simulink library "HORTISIM"  (R2021a)
settings: Solver=VariableStepAuto  StartTime=0.0  StopTime=10.0  RelTol=1e-3
undefined symbols (not defined in the file or in its folder): crop_params, heat_ic, heat_p, p_climate, params_fruit, scr_p, substrate_params, tp_tilapia, win_p, x0_climate, x0_crop, x0_fruit, x0_substrate, x0_tank_tilapia
libraries: $bdroot x10
(part 3 of 4)

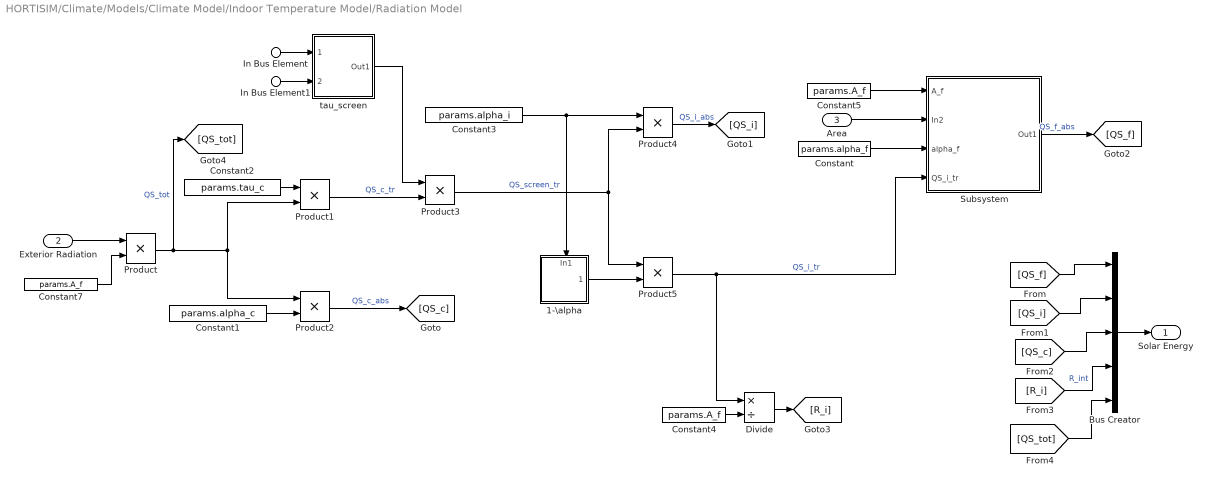
== system HORTISIM/Climate/Models/Climate Model/Indoor Temperature Model/Radiation Model ==
  In Bus Element : Inport  PortName=screen  Element=gamma_max
  In Bus Element1 : Inport  PortName=screen  Element=value
  Exterior Radiation : Inport  Port=2
  Area : Inport  Port=3
  1-\alpha : Subsystem
      settings: PortSchema="{\"entries\":[{\"content\":{\"sides\":[{\"content\":{\"connectorIds\":[]},\"type\":\"ConnectorPlacement.EquallySpacedRectSide\",\"uuid\":\"bf116baa-1c91-42ba-b5ce-6949a5122443\"},{\"content\":{\"connectorIds\":[\"Out1\"],\"side\":\"RIGHT\"},\"type\":\"ConnectorPlacement.EquallySpacedRectSide\",\"uuid\":\"479b2a41-aae8-4d0f-95ce-40d0c52850dd\"},{\"content\":{\"connectorIds\":[\"In1\"],\"side\":\"TOP\"},\"type\":\"ConnectorPlacement.EquallySpacedRectSide\",\"uuid\":\"d0364cd7-422a-4274-8084-cbaa88b34f4b\"}]},\"type\":\"ConnectorPlacement.EquallySpacedConnector\",\"uuid\":\"3d8ba820-72ed-4082-b0d9-d7ce7398093f\"}],\"packageUris\":[\"http://schema.mathworks.com/mf0/Connector/R2020b\"],\"version\":\"1.0\"}"
  Bus Creator : BusCreator  Inputs=5
  Constant : Constant  Value=params.alpha_f
  Constant1 : Constant  Value=params.alpha_c
  Constant2 : Constant  Value=params.tau_c
  Constant3 : Constant  Value=params.alpha_i
  Constant4 : Constant  Value=params.A_f
  Constant5 : Constant  Value=params.A_f
  Constant7 : Constant  Value=params.A_f
  Divide : Product  Inputs=*/
  Product{,1..5} (6 alike) : Product
  Subsystem : Subsystem
  tau_screen : Subsystem
  "Solar Energy  " : Outport
  wires:
  In Bus Element/1 -> tau_screen/1(gamma)
  In Bus Element1/1 -> tau_screen/2(screen)
  [QS_tot] -> Bus Creator/5
  [QS_i] -> Bus Creator/2
  [QS_f] -> Bus Creator/1
  Bus Creator/1 -> "Solar Energy  "/1
  [QS_c] -> Bus Creator/3
  [R_i] -> Bus Creator/4  "R_int"
  Exterior Radiation/1 -> Product/1
  Constant7/1 -> Product/2
  Product/1 -> Product2/1, Product1/2, [QS_tot]  "QS_tot"
  Constant2/1 -> Product1/1
  Constant1/1 -> Product2/2
  Product1/1 -> Product3/2  "QS_c_tr"
  Product2/1 -> [QS_c]  "QS_c_abs"
  tau_screen/1(Out1) -> Product3/1
  Product3/1 -> Product4/2, Product5/1  "QS_screen_tr"
  Constant3/1 -> Product4/1, 1-\alpha/1(In1)
  1-\alpha/1(Out1) -> Product5/2
  Product4/1 -> [QS_i]  "QS_i_abs"
  Constant5/1 -> Subsystem/1(A_f)
  Area/1 -> Subsystem/2(In2)
  Constant/1 -> Subsystem/3(alpha_f)
  Product5/1 -> Subsystem/4(QS_i_tr), Divide/1  "QS_i_tr"
  Subsystem/1(Out1) -> [QS_f]  "QS_f_abs"
  Constant4/1 -> Divide/2
  Divide/1 -> [R_i]

== system HORTISIM/Climate/Models/Climate Model/Indoor Temperature Model/Subsystem ==
  Tc : Inport
  Te : Inport  Port=2
  " Stefan-Boltzmann constant [W/m^2/K^4] " : Constant  Value=5.67e-8
  Bus Creator : BusCreator  Inputs=1
  Constant : Constant  Value=4
  Constant1 : Constant  Value=4
  Constant2 : Constant  Value=params.A_c
  Minus : Sum  Inputs=+-
  Product : Product  Inputs=4
  Square : Math  Operator=pow  SaturateOnIntegerOverflow=on
  Square1 : Math  Operator=pow  SaturateOnIntegerOverflow=on
  k : Constant  Value=0.985
  QR : Outport
  wires:
  Tc/1 -> Square/1
  Constant/1 -> Square/2
  Te/1 -> Square1/1
  Square/1 -> Minus/1
  Square1/1 -> Minus/2
  Constant2/1 -> Product/2
  Minus/1 -> Product/1
  k/1 -> Product/3
  " Stefan-Boltzmann constant [W/m^2/K^4] "/1 -> Product/4
  Constant1/1 -> Square1/2
  Product/1 -> Bus Creator/1  "QR_c_e"
  Bus Creator/1 -> QR/1

== system HORTISIM/Horticulture/Controls/Ferrtirrigation Controler/Irrigation Controler/If Action Subsystem ==
  In1 : Inport
  Action Port : ActionPort
  Constant : Constant
  If : If  IfExpression=u1 > 0.5
  If Action Subsystem : Subsystem  TreatAsAtomicUnit=on
  If Action Subsystem1 : Subsystem  TreatAsAtomicUnit=on
  Merge : Merge
  Mod : Math  Operator=mod  SaturateOnIntegerOverflow=on
  Out1 : Outport
  wires:
  In1/1 -> Mod/1
  Constant/1 -> Mod/2
  Mod/1 -> If/1
  If/1 -> If Action Subsystem/Action
  If/2 -> If Action Subsystem1/Action
  If Action Subsystem/1(Out1) -> Merge/1
  If Action Subsystem1/1(Out1) -> Merge/2
  Merge/1 -> Out1/1

== system HORTISIM/Horticulture/Controls/Ferrtirrigation Controler/Irrigation Controler/If Action Subsystem1 ==
  Action Port : ActionPort
  Constant : Constant  Value=0
  Out1 : Outport
  wires:
  Constant/1 -> Out1/1

== system HORTISIM/Horticulture/Models/Crop Grow/Air Convection/Subsystem ==
  T_i : Inport
  LAI : Inport  Port=2
  T_v : Inport  Port=3
  " characteristic leaf length [m]" : Constant  Value=0.5
  " characteristic leaf length [m]1" : Constant  Value=0.5
  Constant : Constant  Value=params.A_v
  Constant3 : Constant  Value=params.int_air_speed
  Convection1 : MATLAB Function  TreatAsAtomicUnit=on
  Raynols : MATLAB Function  TreatAsAtomicUnit=on
  QV_v_i : Outport
  HV : Outport  Port=2
  wires:
  Constant3/1 -> Raynols/4(int_air_speed)
  " characteristic leaf length [m]1"/1 -> Raynols/3(d_v)
  " characteristic leaf length [m]"/1 -> Convection1/6(d_v)
  Constant/1 -> Convection1/5(A_v)
  Convection1/2(HV) -> HV/1
  Convection1/1(QV_v_i) -> QV_v_i/1
  LAI/1 -> Convection1/4(LAI)
  Raynols/1(Nu) -> Convection1/2(Nu)
  T_i/1 -> [T_i]
  T_v/1 -> [T_v]
  [T_i] -> Raynols/1(T_i)
  [T_v] -> Raynols/2(T_v)
  [T_v] -> Convection1/3(T_v)
  [T_i] -> Convection1/1(T_i)

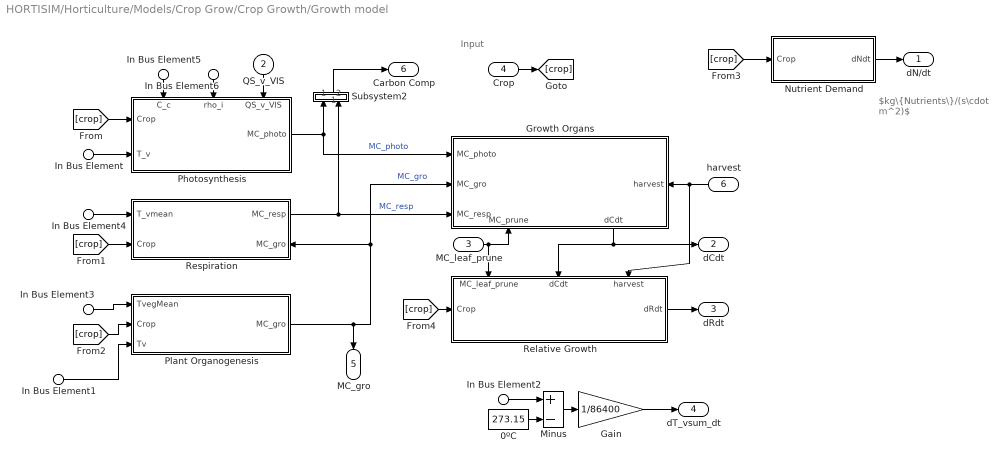
== system HORTISIM/Horticulture/Models/Crop Grow/Crop Growth/Growth model ==
  note: Input
  note: $kg\{Nutrients\}/(s\cdot m^2)$
  In Bus Element5 : Inport  PortName=Gas  Element=C_c
  In Bus Element6 : Inport  PortName=Gas  Element=rho_i
  QS_v_VIS : Inport  Port=2
  MC_leaf_prune : Inport  Port=3
  Crop : Inport  Port=4
  In Bus Element : Inport  Port=5  PortName=Temperature  Element=Tveg
  In Bus Element1 : Inport  Port=5  PortName=Temperature  Element=Tveg
  In Bus Element2 : Inport  Port=5  PortName=Temperature  Element=TvegMean
  In Bus Element3 : Inport  Port=5  PortName=Temperature  Element=TvegMean
  In Bus Element4 : Inport  Port=5  PortName=Temperature  Element=TvegMean
  harvest : Inport  Port=6
  0ºC : Constant  Value=273.15
  Gain : Gain  Gain=1/86400
  Growth Organs : Subsystem
      settings: PortSchema="{\"entries\":[{\"content\":{\"sides\":[{\"content\":{\"connectorIds\":[\"In1\",\"In2\",\"In3\"]},\"type\":\"ConnectorPlacement.EquallySpacedRectSide\",\"uuid\":\"7ed23e67-f8bd-49ca-8750-2aec234a11ce\"},{\"content\":{\"connectorIds\":[\"In5\"],\"side\":\"RIGHT\"},\"type\":\"ConnectorPlacement.EquallySpacedRectSide\",\"uuid\":\"f57cc0dd-0cae-4ca4-a753-4e977147df3f\"},{\"content\":{\"connectorIds\":[],\"side\":\"TOP\"},\"type\":\"ConnectorPlacement.EquallySpacedRectSide\",\"uuid\":\"d3c6828c-1180-4cce-a803-c671dde62607\"},{\"content\":{\"connectorIds\":[\"In4\",\"Out1\"],\"side\":\"BOTTOM\"},\"type\":\"ConnectorPlacement.EquallySpacedRectSide\",\"uuid\":\"2964c671-ea65-49a5-9ed5-5f63619ae496\"}]},\"type\":\"ConnectorPlacement.EquallySpacedConnector\",\"uuid\":\"bc9ae77a-f1c5-46db-8e36-de23e641654c\"}],\"packageUris\":[\"http://schema.mathworks.com/mf0/Connector/R2020b\"],\"version\":\"1.0\"}"
  Minus : Sum  Inputs=+-
  Nutrient Demand : Subsystem
  Photosynthesis : Subsystem
      settings: PortSchema="{\"entries\":[{\"content\":{\"sides\":[{\"content\":{\"connectorIds\":[\"In1\",\"In2\"]},\"type\":\"ConnectorPlacement.EquallySpacedRectSide\",\"uuid\":\"5b7a12d1-e704-4d87-b94c-50c3f7e76c3e\"},{\"content\":{\"connectorIds\":[\"Out1\"],\"side\":\"RIGHT\"},\"type\":\"ConnectorPlacement.EquallySpacedRectSide\",\"uuid\":\"e5762904-c2a4-4288-9297-1f99c7dcb7bb\"},{\"content\":{\"connectorIds\":[\"In3\",\"In4\",\"In5\"],\"side\":\"TOP\"},\"type\":\"ConnectorPlacement.EquallySpacedRectSide\",\"uuid\":\"fedab1c2-3464-4f47-b4b1-20ddf7d17418\"}]},\"type\":\"ConnectorPlacement.EquallySpacedConnector\",\"uuid\":\"14a5d793-cc69-402c-a7d9-30d5c1b3824b\"}],\"packageUris\":[\"http://schema.mathworks.com/mf0/Connector/R2020b\"],\"version\":\"1.0\"}"
  "Plant Organogenesis " : Subsystem
  Relative Growth : Subsystem
      settings: PortSchema="{\"entries\":[{\"content\":{\"sides\":[{\"content\":{\"connectorIds\":[\"In1\"]},\"type\":\"ConnectorPlacement.EquallySpacedRectSide\",\"uuid\":\"3e921aa3-9028-45b3-8678-341874ae1dcc\"},{\"content\":{\"connectorIds\":[\"Out1\"],\"side\":\"RIGHT\"},\"type\":\"ConnectorPlacement.EquallySpacedRectSide\",\"uuid\":\"adeb12d0-e664-4860-aef8-c98149dc4c78\"},{\"content\":{\"connectorIds\":[\"In2\",\"In3\",\"In4\"],\"side\":\"TOP\"},\"type\":\"ConnectorPlacement.EquallySpacedRectSide\",\"uuid\":\"924e6078-7156-46d2-895a-2b088f75d5d0\"}]},\"type\":\"ConnectorPlacement.EquallySpacedConnector\",\"uuid\":\"ff0ec996-f79e-4632-97b2-da63dcaaf854\"}],\"packageUris\":[\"http://schema.mathworks.com/mf0/Connector/R2020b\"],\"version\":\"1.0\"}"
  Respiration : Subsystem
      settings: PortSchema="{\"entries\":[{\"content\":{\"sides\":[{\"content\":{\"connectorIds\":[\"In1\",\"In2\"]},\"type\":\"ConnectorPlacement.EquallySpacedRectSide\",\"uuid\":\"19bf8cd8-dcbb-428b-83dd-ef33216cf6f8\"},{\"content\":{\"connectorIds\":[\"Out1\",\"In3\"],\"side\":\"RIGHT\"},\"type\":\"ConnectorPlacement.EquallySpacedRectSide\",\"uuid\":\"fd2cf296-b399-40a0-bec1-532ab308bb18\"},{\"content\":{\"connectorIds\":[],\"side\":\"TOP\"},\"type\":\"ConnectorPlacement.EquallySpacedRectSide\",\"uuid\":\"43765028-08a6-45c9-8633-a0d1e070a8d0\"}]},\"type\":\"ConnectorPlacement.EquallySpacedConnector\",\"uuid\":\"d52fc605-80b9-4c52-aaab-d44015b38037\"}],\"packageUris\":[\"http://schema.mathworks.com/mf0/Connector/R2020b\"],\"version\":\"1.0\"}"
  Subsystem2 : Subsystem
  dN/dt : Outport
  dCdt : Outport  Port=2
  dRdt : Outport  Port=3
  dT_vsum_dt : Outport  Port=4
  MC_gro : Outport  Port=5
  "Carbon Comp   " : Outport  Port=6
  wires:
  Minus/1 -> Gain/1
  0ºC/1 -> Minus/2
  In Bus Element2/1 -> Minus/1
  Relative Growth/1(dRdt) -> dRdt/1
  Respiration/1(MC_resp) -> Subsystem2/2("         "), Growth Organs/3(MC_resp)  "MC_resp"
  Subsystem2/1("   ") -> "Carbon Comp   "/1
  Gain/1 -> dT_vsum_dt/1
  In Bus Element5/1 -> Photosynthesis/3("C_c ")
  Photosynthesis/1(MC_photo) -> Subsystem2/1(" "), Growth Organs/1(MC_photo)  "MC_photo"
  QS_v_VIS/1 -> Photosynthesis/5(QS_v_VIS)
  "Plant Organogenesis "/1(MC_gro) -> MC_gro/1, Growth Organs/2(MC_gro), Respiration/3(MC_gro)  "MC_gro"
  MC_leaf_prune/1 -> Growth Organs/4(MC_prune), Relative Growth/2(MC_leaf_prune)
  In Bus Element/1 -> Photosynthesis/2(" T_v")
  In Bus Element3/1 -> "Plant Organogenesis "/1(TvegMean)
  Crop/1 -> [crop]
  [crop] -> Photosynthesis/1(Crop)
  [crop] -> Respiration/2(Crop)
  [crop] -> "Plant Organogenesis "/2(Crop)
  [crop] -> Relative Growth/1(Crop)
  In Bus Element4/1 -> Respiration/1(T_vmean)
  In Bus Element6/1 -> Photosynthesis/4(rho_i)
  Nutrient Demand/1(dNdt) -> dN/dt/1
  Growth Organs/1(dCdt) -> dCdt/1, Relative Growth/3(dCdt)
  [crop] -> Nutrient Demand/1(Crop)
  harvest/1 -> Relative Growth/4(harvest), Growth Organs/5(harvest)
  In Bus Element1/1 -> "Plant Organogenesis "/3(Tv)

== system HORTISIM/Horticulture/Models/Crop Grow/Crop Growth/Subsystem ==
  In1 : Inport
  Bus Creator : BusCreator  Inputs=4
  Demux : Demux
  Out1 : Outport
  wires:
  In1/1 -> Demux/1
  Demux/1 -> Bus Creator/1  "Cbuff"
  Demux/2 -> Bus Creator/2  "Cfruit"
  Demux/3 -> Bus Creator/3  "Cleaf"
  Demux/4 -> Bus Creator/4  "Cstem"
  Bus Creator/1 -> Out1/1

== system HORTISIM/Horticulture/Models/Crop Grow/Crop Growth/Subsystem1 ==
  In1 : Inport
  Bus Creator : BusCreator  Inputs=3
  Demux : Demux  Outputs=3
  Out1 : Outport
  wires:
  In1/1 -> Demux/1
  Demux/1 -> Bus Creator/1  "Rfruit"
  Demux/2 -> Bus Creator/2  "Rleaf"
  Demux/3 -> Bus Creator/3  "Rstem"
  Bus Creator/1 -> Out1/1

== system HORTISIM/Horticulture/Models/Crop Grow/Crop Growth/Subsystem2 ==
  M : Inport
  ND : Inport  Port=2
  Bus Creator : BusCreator  Inputs=2
  Out1 : Outport
  wires:
  ND/1 -> Bus Creator/2  "Demand"
  M/1 -> Bus Creator/1  "Mass"
  Bus Creator/1 -> Out1/1

== system HORTISIM/Horticulture/Models/Crop Grow/Merges/Subsystem ==
  note: $kg\{C\}/m^2$
  note: $kg\{H_2O\}/kg\{C\}$
  note: $kg\{H_2O\}/m^2$
  note: $kg\{H_2O\}/m^2$
  note: $kg\{H_2O\}/m^2$
  Ctot : Inport
  Constant4 : Constant  Value=params.min_water_capacity
  Convertion Ratio : Subsystem
  Product : Product
  Sum : Sum  Inputs=|++
  WaterCapacity : Outport
  wires:
  Ctot/1 -> Product/1
  Product/1 -> Sum/1
  Constant4/1 -> Sum/2
  Sum/1 -> WaterCapacity/1
  Convertion Ratio/1(Out1) -> Product/2

== system HORTISIM/Horticulture/Models/Crop Grow/Merges/Subsystem1 ==
  note: $kg\{H_2O\}/m^2$
  note: $kg\{H_2O\}/m^2$
  WC : Inport
  C_wv : Inport  Port=2
  Divide : Product  Inputs=*/
  WaterPercent : Outport
  wires:
  C_wv/1 -> Divide/1
  WC/1 -> Divide/2
  Divide/1 -> WaterPercent/1

== system HORTISIM/Horticulture/Models/Crop Grow/Merges/Subsystem2 ==
  In1 : Inport
  " molar mass of CH2O [kg/mol]" : Constant  Value=0.03
  Bus Selector1 : BusSelector  OutputSignals=MC_i_buf,MC_buf_i,MC_fruit_i,MC_leaf_i,MC_stem_i
  Constant2 : Constant  Value=params.A_v
  Divide : Product  Inputs=*/**
  Sum1 : Sum  Inputs=|-++++
  molar mass of CO2 [kg/mol] : Constant  Value=0.044
  MC_v_i : Outport
  wires:
  Bus Selector1/4 -> Sum1/4  "<MC_leaf_i>"
  Bus Selector1/3 -> Sum1/3  "<MC_fruit_i>"
  In1/1 -> Bus Selector1/1
  molar mass of CO2 [kg/mol]/1 -> Divide/1
  Constant2/1 -> Divide/3
  Divide/1 -> MC_v_i/1  "MC_v_i"
  Bus Selector1/2 -> Sum1/2  "<MC_buf_i>"
  Sum1/1 -> Divide/4
  " molar mass of CH2O [kg/mol]"/1 -> Divide/2
  Bus Selector1/5 -> Sum1/5  "<MC_stem_i>"
  Bus Selector1/1 -> Sum1/1  "<MC_i_buf>"

== system HORTISIM/Horticulture/Models/Crop Grow/Subsystem/Subsystem ==
  <LAI> : Inport
  Constant : Constant  Value=0.95
  Exp : Math  SaturateOnIntegerOverflow=on
  Gain : Gain  Gain=-1
  Gain1 : Gain  Gain=0.9
  Product : Product
  Sum : Sum  Inputs=|+-
  Visible diffuse extinction coefficient [-] : Constant  Value=0.85
  Out1 : Outport
  wires:
  Exp/1 -> Gain1/1
  <LAI>/1 -> Product/1
  Sum/1 -> Out1/1
  Gain1/1 -> Sum/2
  Product/1 -> Gain/1
  Gain/1 -> Exp/1
  Constant/1 -> Sum/1
  Visible diffuse extinction coefficient [-]/1 -> Product/2

== system HORTISIM/Horticulture/Models/Crop Grow/Subsystem/Subsystem1 ==
  <LAI> : Inport
  Constant : Constant  Value=0.95
  Exp : Math  SaturateOnIntegerOverflow=on
  Gain : Gain  Gain=-1
  Gain1 : Gain  Gain=0.9
  Product : Product
  Sum : Sum  Inputs=|+-
  Visible diffuse extinction coefficient [-] : Constant  Value=0.5
  Out1 : Outport
  wires:
  Exp/1 -> Gain1/1
  <LAI>/1 -> Product/1
  Sum/1 -> Out1/1
  Gain1/1 -> Sum/2
  Product/1 -> Gain/1
  Gain/1 -> Exp/1
  Constant/1 -> Sum/1
  Visible diffuse extinction coefficient [-]/1 -> Product/2

== system HORTISIM/Horticulture/Models/Crop Grow/Transpiration/Subsystem1 ==
  C_w : Inport
  rho_i : Inport  Port=2
  T_v : Inport  Port=3
  Constant : Constant  Value=0.622
  Divide : Product  Inputs=*/
  Divide1 : Product  Inputs=/*
  Divide2 : Product  Inputs=*/
  Divide3 : Product  Inputs=*/
  Minus : Sum  Inputs=-+
  Product : Product
  Sum : Sum  Inputs=|++
  Sum1 : Sum  Inputs=|++
  Temp2SatDensity : $bdroot/Other  Functions/Temp2SatDensity  SystemSampleTime=-1  VariantActivationTime=update diagram  Latency=0  AutoFrameSizeCalculation=off
  atm : Constant  Value=101300
  vpd : Outport
  wires:
  Product/1 -> vpd/1  "vpd"
  C_w/1 -> Divide/1
  T_v/1 -> Temp2SatDensity/1
  Temp2SatDensity/1 -> Divide1/2
  rho_i/1 -> Divide1/1, Divide/2
  Divide1/1 -> Divide3/1, Sum1/2  "xv"
  Constant/1 -> Sum1/1, Sum/2
  Divide/1 -> Divide2/1, Sum/1  "xa"
  Sum/1 -> Divide2/2
  Sum1/1 -> Divide3/2
  Divide2/1 -> Minus/1
  Divide3/1 -> Minus/2
  Minus/1 -> Product/2
  atm/1 -> Product/1

== system HORTISIM/Horticulture/Models/Crop Grow/Water Balance/Subsystem ==
  Real Water Uptake : Inport
  Evapotranspiration : Inport  Port=2
  Gain8 : Gain  Gain=24*3600
  Sum : Sum  Inputs=|+-
  Water Content : Integrator  InitialCondition=x0.C_wv  AbsoluteTolerance=1e-3
  C_wv : Outport
  wires:
  Evapotranspiration/1 -> Sum/2
  Sum/1 -> Gain8/1
  Water Content/1 -> C_wv/1  "C_wv"
  Real Water Uptake/1 -> Sum/1
  Gain8/1 -> Water Content/1

== system HORTISIM/Horticulture/Models/Crop Grow/Water Balance/Subsystem1 ==
  note: $kg\{H_2O\}/m^2$
  note: $1/s$
  <WaterPercent> : Inport
  <WC> : Inport  Port=2
  " " : Gain  Gain=5e-1
  Constant : Constant  Value=0.95
  Constant1 : Constant  Value=0
  Gain : Gain  Gain=1/100
  Max : MinMax  Function=max  Inputs=2
  Minus : Sum  Inputs=+-
  Product : Product
  Out1 : Outport
  wires:
  <WaterPercent>/1 -> Minus/2
  Minus/1 -> Gain/1
  Product/1 -> " "/1
  Constant/1 -> Minus/1
  " "/1 -> Max/1
  Constant1/1 -> Max/2
  Max/1 -> Out1/1
  <WC>/1 -> Product/2
  Gain/1 -> Product/1

== system HORTISIM/Horticulture/Models/Substrate Bag/Nutrient Balance/Subsystem ==
  V : Inport
  Mass : Inport  Port=2
  Bus Selector : BusSelector  OutputSignals=VT
  Divide : Product  Inputs=*/
  X : Outport
  wires:
  Divide/1 -> X/1  "X"
  Mass/1 -> Divide/1
  V/1 -> Bus Selector/1
  Bus Selector/1 -> Divide/2  "<VT>"

== system HORTISIM/Horticulture/Models/Substrate Bag/Nutrient Balance/Subsystem1 ==
  Demand : Inport
  Content : Inport  Port=2
  Constant1 : Constant  Value=0.5
  Constant2 : Constant  Value=params.Nmin_subs
  Gain : Gain  Gain=10
  Gain3 : Gain  Gain=0.5
  Minus1 : Sum  Inputs=+-
  Product : Product
  Sum1 : Sum  Inputs=|++
  Tanh : Trigonometry  Operator=tanh
  RealNutrientUptake : Outport
  wires:
  Tanh/1 -> Gain3/1
  Constant1/1 -> Sum1/2
  Gain3/1 -> Sum1/1
  Gain/1 -> Tanh/1
  Constant2/1 -> Minus1/2
  Minus1/1 -> Gain/1
  Sum1/1 -> Product/2
  Content/1 -> Minus1/1
  Product/1 -> RealNutrientUptake/1
  Demand/1 -> Product/1

== system HORTISIM/Horticulture/Models/Substrate Bag/Subsystem3/V0 ==
  fin : Inport
  Demand : Inport  Port=2
  Gain : Gain  Gain=1e-3
  Gain1 : Gain  Gain=24*3600
  Product : Product
  Subsystem : Subsystem
  Subsystem1 : Subsystem
  Sum1 : Sum  Inputs=-+--
  Water Substrate Level 0 : Integrator  InitialCondition=x0.C_ws  AbsoluteTolerance=1e-3
  rho : Gain  Gain=5e-3
  V : Outport
  f_out : Outport  Port=2
  d_out : Outport  Port=3
  WaterUptake : Outport  Port=4
  wires:
  fin/1 -> Sum1/2
  Gain1/1 -> Water Substrate Level 0/1
  Water Substrate Level 0/1 -> [V], rho/1, V/1  "C_ws"
  rho/1 -> f_out/1, Sum1/3
  Sum1/1 -> Gain1/1
  [V] -> Subsystem/1(V)
  [V] -> Subsystem1/1(V)
  Subsystem1/1(Out1) -> Product/2
  Product/1 -> WaterUptake/1, Sum1/1
  Demand/1 -> Product/1
  Subsystem/1(Out1) -> Gain/1
  Gain/1 -> d_out/1, Sum1/4

== system HORTISIM/Horticulture/Models/Substrate Bag/Subsystem3/V1 ==
  fin : Inport
  Demand : Inport  Port=2
  Gain : Gain  Gain=1e-3
  Gain1 : Gain  Gain=24*3600
  Product : Product
  Subsystem : Subsystem
  Subsystem1 : Subsystem
  Sum1 : Sum  Inputs=-+--
  Water Substrate Level 0 : Integrator  InitialCondition=x0.C_ws  AbsoluteTolerance=1e-3
  rho : Gain  Gain=5e-3
  V : Outport
  f_out : Outport  Port=2
  d_out : Outport  Port=3
  WaterUptake : Outport  Port=4
  wires:
  fin/1 -> Sum1/2
  Gain1/1 -> Water Substrate Level 0/1
  Water Substrate Level 0/1 -> [V], rho/1, V/1  "C_ws"
  rho/1 -> f_out/1, Sum1/3
  Sum1/1 -> Gain1/1
  [V] -> Subsystem/1(V)
  [V] -> Subsystem1/1(V)
  Subsystem1/1(Out1) -> Product/2
  Product/1 -> WaterUptake/1, Sum1/1
  Demand/1 -> Product/1
  Subsystem/1(Out1) -> Gain/1
  Gain/1 -> d_out/1, Sum1/4

== system HORTISIM/Horticulture/Models/Substrate Bag/Subsystem3/V2 ==
  fin : Inport
  Demand : Inport  Port=2
  Gain : Gain  Gain=1e-3
  Gain1 : Gain  Gain=24*3600
  Product : Product
  Subsystem : Subsystem
  Subsystem1 : Subsystem
  Sum1 : Sum  Inputs=-+--
  Water Substrate Level 0 : Integrator  InitialCondition=x0.C_ws  AbsoluteTolerance=1e-3
  rho : Gain  Gain=5e-3
  V : Outport
  f_out : Outport  Port=2
  d_out : Outport  Port=3
  WaterUptake : Outport  Port=4
  wires:
  fin/1 -> Sum1/2
  Gain1/1 -> Water Substrate Level 0/1
  Water Substrate Level 0/1 -> [V], rho/1, V/1  "C_ws"
  rho/1 -> f_out/1, Sum1/3
  Sum1/1 -> Gain1/1
  [V] -> Subsystem/1(V)
  [V] -> Subsystem1/1(V)
  Subsystem1/1(Out1) -> Product/2
  Product/1 -> WaterUptake/1, Sum1/1
  Demand/1 -> Product/1
  Subsystem/1(Out1) -> Gain/1
  Gain/1 -> d_out/1, Sum1/4

== system HORTISIM/Aquaculture/Models/Tank Model/Heat Balances/Convection Air 2 Water Tanl Surface/Gr ==
  d : Inport
  T_air : Inport  Port=2
  T_w : Inport  Port=3
  Abs : Abs
  Constant : Constant  Value=3
  Constant1 : Constant  Value=1/(1.5100e-05)^2
  Divide : Product  Inputs=*/
  Minus : Sum  Inputs=+-
  Pow : Math  Operator=pow  SignedPower=on  RndMeth=Zero  SaturateOnIntegerOverflow=on
  Product : Product  Inputs=4
  g [m/s^2] : Constant  Value=9.8
  Gr : Outport
  wires:
  T_air/1 -> Divide/2, Minus/1
  T_w/1 -> Minus/2
  Minus/1 -> Abs/1
  Abs/1 -> Divide/1
  d/1 -> Pow/1
  Constant/1 -> Pow/2
  Divide/1 -> Product/2
  g [m/s^2]/1 -> Product/1
  Pow/1 -> Product/3
  Constant1/1 -> Product/4
  Product/1 -> Gr/1

== system HORTISIM/Aquaculture/Models/Tank Model/Heat Balances/Convection Air 2 Water Tanl Surface/Gr2vG ==
  Gr : Inport
  Constant : Constant  Value=0.25
  If : If  IfExpression=u1 < 1e5
  If Action Subsystem : Subsystem  TreatAsAtomicUnit=on
  If Action Subsystem1 : Subsystem  TreatAsAtomicUnit=on
  "Le = 0.8190; % Lewis number [-] " : Constant  Value=0.8190
  Merge : Merge
  Pow : Math  Operator=pow  SignedPower=on  RndMeth=Zero  SaturateOnIntegerOverflow=on
  Product : Product
  Out1 : Outport
  Out2 : Outport  Port=2
  wires:
  Gr/1 -> If Action Subsystem1/1(Gr), If Action Subsystem/1(Gr), If/1
  If/1 -> If Action Subsystem/Action
  If/2 -> If Action Subsystem1/Action
  If Action Subsystem/1(Out1) -> Merge/1
  If Action Subsystem1/1(Out1) -> Merge/2
  Merge/1 -> Product/1, Out1/1
  Product/1 -> Out2/1
  "Le = 0.8190; % Lewis number [-] "/1 -> Pow/1
  Pow/1 -> Product/2
  Constant/1 -> Pow/2

== system HORTISIM/Aquaculture/Models/Tank Model/Heat Balances/Convection Air 2 Water Tanl Surface/Re ==
  d_w : Inport
  wind_speed : Inport  Port=2
  Divide : Product  Inputs=**/
  kinematic viscosity [m^2/s] : Constant  Value=1.5100e-05
  Re : Outport
  wires:
  d_w/1 -> Divide/1
  wind_speed/1 -> Divide/2
  kinematic viscosity [m^2/s]/1 -> Divide/3
  Divide/1 -> Re/1

== system HORTISIM/Aquaculture/Models/Tank Model/Heat Balances/Convection Air 2 Water Tanl Surface/Re2vR ==
  Re : Inport
  Constant : Constant  Value=0.33
  If : If  IfExpression=u1 < 2e4
  If Action Subsystem : Subsystem  TreatAsAtomicUnit=on
  If Action Subsystem1 : Subsystem  TreatAsAtomicUnit=on
  "Le = 0.8190; % Lewis number [-] " : Constant  Value=0.8190
  Merge : Merge
  Pow : Math  Operator=pow  SignedPower=on  RndMeth=Zero  SaturateOnIntegerOverflow=on
  Product : Product
  Out1 : Outport
  Out2 : Outport  Port=2
  wires:
  Re/1 -> If Action Subsystem1/1(Re), If Action Subsystem/1(Re), If/1
  If/1 -> If Action Subsystem/Action
  If/2 -> If Action Subsystem1/Action
  If Action Subsystem/1(Out1) -> Merge/1
  If Action Subsystem1/1(Out1) -> Merge/2
  Merge/1 -> Product/1, Out1/1
  "Le = 0.8190; % Lewis number [-] "/1 -> Pow/1
  Constant/1 -> Pow/2
  Pow/1 -> Product/2
  Product/1 -> Out2/1

== system HORTISIM/Aquaculture/Models/Tank Model/Heat Balances/Convection Air 2 Water Tanl Surface/Subsystem ==
  In1 : Inport
  In2 : Inport  Port=2
  In3 : Inport  Port=3
  In4 : Inport  Port=4
  If : If  NumInputs=2  IfExpression=u1 > u2
  If Action Subsystem : Subsystem  TreatAsAtomicUnit=on
  If Action Subsystem1 : Subsystem  TreatAsAtomicUnit=on
  Merge : Merge
  Merge1 : Merge
  nu : Outport
  sh : Outport  Port=2
  wires:
  Merge1/1 -> nu/1  "nu"
  In4/1 -> If Action Subsystem1/2(In2)
  If Action Subsystem1/2(Out2) -> Merge/2
  In3/1 -> If Action Subsystem1/1(In1), If/2
  If/1 -> If Action Subsystem/Action
  If Action Subsystem/2(Out2) -> Merge/1
  Merge/1 -> sh/1  "sh"
  If Action Subsystem/1(Out1) -> Merge1/1
  If Action Subsystem1/1(Out1) -> Merge1/2
  In1/1 -> If Action Subsystem/1(In1), If/1
  In2/1 -> If Action Subsystem/2(In2)
  If/2 -> If Action Subsystem1/Action

== system HORTISIM/Aquaculture/Models/Tank Model/Heat Balances/Transpiration/Ratio of Humidity Sat ==
  T : Inport
  p_a : Inport  Port=2
  Divide2 : Product  Inputs=*/
  Gain1 : Gain  Gain=0.62198
  MATLAB Function : MATLAB Function  TreatAsAtomicUnit=on
  Minus : Sum  Inputs=+-
  Scope : Scope  NumInputPorts=2
  Out1 : Outport
  wires:
  p_a/1 -> Minus/1, Scope/2
  Minus/1 -> Divide2/2
  Gain1/1 -> Out1/1
  MATLAB Function/1(r) -> Divide2/1, Minus/2, Scope/1  "p_w^*"
  Divide2/1 -> Gain1/1
  T/1 -> MATLAB Function/1(T)

== system HORTISIM/Aquaculture/Models/Tank Model/Subsystem/Subsystem1/For Each Subsystem ==
  Fin : Inport  Partition=on  PartitionDimension=1  PartitionWidth=1  PartitionOffset=0
  X : Inport  Port=2
  Bus Selector : BusSelector  OutputSignals=f,X,T
  For Each : ForEach  DisableCoverage=on
  If : If
  If Action Subsystem : Subsystem  TreatAsAtomicUnit=on
  If Action Subsystem1 : Subsystem  TreatAsAtomicUnit=on
  Merge : Merge
  fs : Outport  ConcatenationDimension=1
  Xs : Outport  Port=2  ConcatenationDimension=2
  T : Outport  Port=3  ConcatenationDimension=1
  wires:
  Bus Selector/3 -> T/1  "<T>"
  Fin/1 -> Bus Selector/1
  Bus Selector/1 -> If/1, fs/1  "<f>"
  Bus Selector/2 -> If Action Subsystem/1(In1)  "<X>"
  If/1 -> If Action Subsystem/Action
  If/2 -> If Action Subsystem1/Action
  X/1 -> If Action Subsystem1/1(X)
  Merge/1 -> Xs/1
  If Action Subsystem/1(Out1) -> Merge/1
  If Action Subsystem1/1(Out1) -> Merge/2

== system HORTISIM/Aquaculture/Models/Tank Model/Subsystem/Subsystem1/For Each Subsystem1 ==
  fs : Inport  Partition=on  PartitionDimension=2  PartitionWidth=1  PartitionOffset=0
  ps : Inport  Port=2  Partition=on  PartitionDimension=2  PartitionWidth=1  PartitionOffset=0
  For Each : ForEach  DisableCoverage=on
  Product : Product
  Out1 : Outport  ConcatenationDimension=2
  wires:
  fs/1 -> Product/1
  ps/1 -> Product/2
  Product/1 -> Out1/1

== system HORTISIM/Aquaculture/Models/Tank Model/Subsystem/Subsystem2/For Each Subsystem ==
  Fin : Inport  Partition=on  PartitionDimension=1  PartitionWidth=1  PartitionOffset=0
  Bus Selector : BusSelector  OutputSignals=f,X,T
  For Each : ForEach  DisableCoverage=on
  fs : Outport  ConcatenationDimension=1
  Xs : Outport  Port=2  ConcatenationDimension=2
  Ts : Outport  Port=3  ConcatenationDimension=2
  wires:
  Bus Selector/3 -> Ts/1  "<T>"
  Fin/1 -> Bus Selector/1
  Bus Selector/1 -> fs/1  "<f>"
  Bus Selector/2 -> Xs/1  "<X>"

== system HORTISIM/Aquaculture/Models/Tank Model/Subsystem/Subsystem2/For Each Subsystem1 ==
  fs : Inport  Partition=on  PartitionDimension=2  PartitionWidth=1  PartitionOffset=0
  ps : Inport  Port=2  Partition=on  PartitionDimension=2  PartitionWidth=1  PartitionOffset=0
  For Each : ForEach  DisableCoverage=on
  Product : Product
  Out1 : Outport  ConcatenationDimension=2
  wires:
  fs/1 -> Product/1
  ps/1 -> Product/2
  Product/1 -> Out1/1

== system HORTISIM/Climate/Controls/Fogging Controler/Subsystem/Subsystem2/If Action Subsystem ==
  Action Port : ActionPort
  Constant : Constant  Value=0
  Out1 : Outport
  wires:
  Constant/1 -> Out1/1

== system HORTISIM/Climate/Controls/Fogging Controler/Subsystem/Subsystem2/If Action Subsystem1 ==
  Action Port : ActionPort
  Constant : Constant
  Out1 : Outport
  wires:
  Constant/1 -> Out1/1

== system HORTISIM/Climate/Controls/Fogging Controler/Subsystem/Subsystem2/If Action Subsystem2 ==
  In1 : Inport
  Action Port : ActionPort
  Out1 : Outport
  wires:
  In1/1 -> Out1/1

== system HORTISIM/Climate/Controls/Heating Controler/Subsystem/Subsystem1/Subsystem ==
  Ti : Inport
  Th : Inport  Port=2
  " nu kinematic viscosity [m^2/s]" : Constant  Value=15.1e-6
  Abs : Abs
  Constant : Constant  Value=3
  Divide : Product  Inputs=*/
  Divide1 : Product  Inputs=*/
  Minus : Sum  Inputs=+-
  Power : Math  Operator=pow  SaturateOnIntegerOverflow=on
  Product : Product
  Product1 : Product
  Square : Math  Operator=square  SaturateOnIntegerOverflow=on
  d_h : Constant  Value=1.5
  g acceleration due to gravity [m/s^2] : Constant  Value=9.81
  Gr : Outport
  dT : Outport  Port=2
  wires:
  Ti/1 -> Minus/2, Divide/2
  Power/1 -> Product/2
  d_h/1 -> Power/1
  Minus/1 -> Abs/1, dT/1
  " nu kinematic viscosity [m^2/s]"/1 -> Square/1
  Th/1 -> Minus/1
  Constant/1 -> Power/2
  Product/1 -> Divide1/1
  Square/1 -> Divide1/2
  Product1/1 -> Gr/1
  Divide/1 -> Product1/2
  Divide1/1 -> Product1/1
  Abs/1 -> Divide/1
  g acceleration due to gravity [m/s^2]/1 -> Product/1

== system HORTISIM/Climate/Controls/Heating Controler/Subsystem/Subsystem2/Subsystem ==
  Ti : Inport
  Th : Inport  Port=2
  " nu kinematic viscosity [m^2/s]" : Constant  Value=15.1e-6
  Abs : Abs
  Constant : Constant  Value=3
  Divide : Product  Inputs=*/
  Divide1 : Product  Inputs=*/
  Minus : Sum  Inputs=+-
  Power : Math  Operator=pow  SaturateOnIntegerOverflow=on
  Product : Product
  Product1 : Product
  Square : Math  Operator=square  SaturateOnIntegerOverflow=on
  d_h : Constant  Value=1.5
  g acceleration due to gravity [m/s^2] : Constant  Value=9.81
  Gr : Outport
  dT : Outport  Port=2
  wires:
  Ti/1 -> Minus/2, Divide/2
  Power/1 -> Product/2
  d_h/1 -> Power/1
  Minus/1 -> Abs/1, dT/1
  " nu kinematic viscosity [m^2/s]"/1 -> Square/1
  Th/1 -> Minus/1
  Constant/1 -> Power/2
  Product/1 -> Divide1/1
  Square/1 -> Divide1/2
  Product1/1 -> Gr/1
  Divide/1 -> Product1/2
  Divide1/1 -> Product1/1
  Abs/1 -> Divide/1
  g acceleration due to gravity [m/s^2]/1 -> Product/1

== system HORTISIM/Climate/Controls/Screen Controler/Subsystem/If Action Subsystem1/Theta  ==
  In1 : Inport
  Constant1 : Constant  Value=0.5
  Gain : Gain  Gain=0.5
  Sign : Signum  ZeroCross=off
  Sum : Sum  Inputs=|++
  Out1 : Outport
  wires:
  Constant1/1 -> Sum/2
  In1/1 -> Sign/1
  Gain/1 -> Sum/1
  Sum/1 -> Out1/1
  Sign/1 -> Gain/1

== system HORTISIM/Climate/Models/Climate Model/Gases Exchange/Carbon Dynamics/Carbon Exchange Indoor-Outdoor ==
  R_a : Inport
  C_c : Inport  Port=2
  C_ce : Inport  Port=3
  Minus : Sum  Inputs=+-
  Product : Product
  MC_i_e : Outport
  wires:
  C_c/1 -> Minus/1
  C_ce/1 -> Minus/2
  Minus/1 -> Product/2
  R_a/1 -> Product/1
  Product/1 -> MC_i_e/1

== system HORTISIM/Climate/Models/Climate Model/Gases Exchange/Carbon Dynamics/External CO2 Concentration ==
  T_e : Inport
  Divide : Product  Inputs=**//
  Gain : Gain  Gain=4e-4
  M_c : Constant  Value=0.0440
  R : Constant  Value=8.3140
  atm : Constant  Value=101300
  C_ce : Outport
  wires:
  atm/1 -> Divide/1
  R/1 -> Divide/3
  M_c/1 -> Divide/2
  T_e/1 -> Divide/4
  Divide/1 -> Gain/1
  Gain/1 -> C_ce/1

== system HORTISIM/Climate/Models/Climate Model/Gases Exchange/Compute Mid Variables/Subsystem ==
  Gas_Conc : Inport
  IndoorTemp : Inport  Port=2
  Air Density : MATLAB Function  TreatAsAtomicUnit=on
  Bus Selector : BusSelector  OutputSignals=Tair,Tcover,Tfloor
  Demux : Demux  Outputs=2
  Divide : Product  Inputs=*/
  Gain : Gain  Gain=100
  Ratio of Humidity Sat : Subsystem
  Temp2SatDensity : $bdroot/Other  Functions/Temp2SatDensity  SystemSampleTime=-1  VariantActivationTime=update diagram  Latency=0  AutoFrameSizeCalculation=off
  Temp2SatDensity1 : $bdroot/Other  Functions/Temp2SatDensity  SystemSampleTime=-1  VariantActivationTime=update diagram  Latency=0  AutoFrameSizeCalculation=off
  Temp2SatDensity2 : $bdroot/Other  Functions/Temp2SatDensity  SystemSampleTime=-1  VariantActivationTime=update diagram  Latency=0  AutoFrameSizeCalculation=off
  rho_i : Outport
  C_c_ppm : Outport  Port=2
  HRInt : Outport  Port=3
  C_w_sat_T_c : Outport  Port=4
  C_w_sat_T_f : Outport  Port=5
  xH : Outport  Port=6
  p_a : Outport  Port=7
  xH_sat : Outport  Port=8
  wires:
  IndoorTemp/1 -> Bus Selector/1
  Bus Selector/1 -> Ratio of Humidity Sat/1(<Tair>), Air Density/3(T_i), Temp2SatDensity2/1  "<Tair>"
  Gas_Conc/1 -> Demux/1
  Bus Selector/2 -> Temp2SatDensity/1  "<Tcover>"
  Bus Selector/3 -> Temp2SatDensity1/1  "<Tfloor>"
  Temp2SatDensity/1 -> C_w_sat_T_c/1
  Temp2SatDensity1/1 -> C_w_sat_T_f/1
  Demux/1 -> [C_w]  "C_w"
  Demux/2 -> Air Density/2(C_c)  "C_c"
  Air Density/1(rho_i) -> rho_i/1
  Air Density/2(C_c_ppm) -> C_c_ppm/1
  [C_w] -> Air Density/1(C_w)
  Air Density/3(xH) -> xH/1
  Air Density/4(p_a) -> Ratio of Humidity Sat/2(p_a), p_a/1
  Temp2SatDensity2/1 -> Ratio of Humidity Sat/3(sat_C_w), Divide/2
  Gain/1 -> Divide/1
  [C_w] -> Gain/1
  Divide/1 -> HRInt/1  "HRInt"
  Ratio of Humidity Sat/1(Out1) -> xH_sat/1

== system HORTISIM/Climate/Models/Climate Model/Gases Exchange/Water Dynamics/Subsystem ==
  <Temperature> : Inport
  <Exterior Humidity> : Inport  Port=2
  Gain : Gain  Gain=1/100
  Product : Product
  Temp2SatDensity : $bdroot/Other  Functions/Temp2SatDensity  SystemSampleTime=-1  VariantActivationTime=update diagram  Latency=0  AutoFrameSizeCalculation=off
  C_w_Te : Outport
  wires:
  Product/1 -> C_w_Te/1  "C_w_Te"
  <Temperature>/1 -> Temp2SatDensity/1
  <Exterior Humidity>/1 -> Gain/1
  Temp2SatDensity/1 -> Product/1  "C_w_sat_Te"
  Gain/1 -> Product/2

== system HORTISIM/Climate/Models/Climate Model/Gases Exchange/Water Dynamics/Vapor Mass Balance ==
  <QT_v_i> : Inport
  <Qfog> : Inport  Port=2
  MW_i_e : Inport  Port=3
  <QP_i_c> : Inport  Port=4
  <QP_i_f> : Inport  Port=5
  Constant1 : Constant  Value=params.V
  Divide : Product  Inputs=*/
  Divide1 : Product  Inputs=*/
  Minus : Sum  Inputs=+-
  Product : Product
  Scope : Scope
  Scope1 : Scope
  Sum : Sum  Inputs=|+--+
  latent heat of condensation of water [J/kg] : Constant  Value=2437000
  dC_w_dt : Outport
  wires:
  latent heat of condensation of water [J/kg]/1 -> Product/1
  Constant1/1 -> Product/2
  <QT_v_i>/1 -> Divide1/1, Sum/1
  <QP_i_c>/1 -> Scope1/1, Sum/2
  <QP_i_f>/1 -> Sum/3
  <Qfog>/1 -> Sum/4
  Sum/1 -> Divide/1
  Product/1 -> Divide1/2, Divide/2
  Divide/1 -> Minus/1
  MW_i_e/1 -> Minus/2
  Minus/1 -> dC_w_dt/1
  Divide1/1 -> Scope/1

== system HORTISIM/Climate/Models/Climate Model/Indoor Temperature Model/Convection/Convection ==
  IndoorTemp : Inport
  Cw_Tc : Inport  Port=2
  Cw_Tf : Inport  Port=3
  T_e : Inport  Port=4
  wind_speed : Inport  Port=5
  rho_i : Inport  Port=6
  C_w : Inport  Port=7
  Bus Creator : BusCreator  Inputs=2
  Bus Selector1 : BusSelector  OutputSignals=Tcover,Tair,Tfloor
  Constant : Constant  Value=0
  Constant1 : Constant  Value=params.A_f
  Constant2 : Constant  Value=params.A_f
  Constant3 : Constant  Value=params.d_c
  Constant4 : Constant  Value=0.5
  Constant5 : Constant  Value=params.int_air_speed
  Convection : MATLAB Function  TreatAsAtomicUnit=on
  Max : MinMax  Function=max  Inputs=2
  Max1 : MinMax  Function=max  Inputs=2
  QV_c_e : Outport
  QV_i_c : Outport  Port=2
  QV_i_f : Outport  Port=3
  QP : Outport  Port=4
  wires:
  Convection/1(QV_c_e) -> QV_c_e/1
  Convection/2(QV_i_c) -> QV_i_c/1
  Convection/3(QV_i_f) -> QV_i_f/1
  Bus Creator/1 -> QP/1
  C_w/1 -> Convection/6(C_w)
  rho_i/1 -> Convection/7(rho_i)
  Constant/1 -> Max1/1, Max/2
  Convection/5(QP_i_f) -> Max1/2
  Convection/4(QP_i_c) -> Max/1
  Max1/1 -> Bus Creator/2  "QP_i_f"
  Max/1 -> Bus Creator/1  "QP_i_c"
  IndoorTemp/1 -> Bus Selector1/1
  Bus Selector1/1 -> Convection/1(T_c)  "<Tcover>"
  Bus Selector1/2 -> Convection/2(T_i)  "<Tair>"
  Bus Selector1/3 -> Convection/3(T_f)  "<Tfloor>"
  T_e/1 -> Convection/4(T_e)
  wind_speed/1 -> Convection/5(wind_speed)
  Constant1/1 -> Convection/8(A_f)
  Constant2/1 -> Convection/9(A_c)
  Constant3/1 -> Convection/10(d_c)
  Constant4/1 -> Convection/11(d_f)
  Constant5/1 -> Convection/12(int_air_speed)
  Cw_Tf/1 -> Convection/14(C_w_sat_T_f)
  Cw_Tc/1 -> Convection/13(C_w_sat_T_c)

== system HORTISIM/Climate/Models/Climate Model/Indoor Temperature Model/Convection/Subsystem ==
  T_e : Inport
  wind_speed : Inport  Port=2
  <Tair> : Inport  Port=3
  In Bus Element1 : Inport  Port=4  PortName=Windows  Element=value
  In Bus Element : Inport  Port=4  PortName=Windows  Element=AR
  rho_i : Inport  Port=5
  AR1 : Constant  Value=params.minWindows  VectorParams1D=off
  Abs : Abs
  Cd : Constant  Value=0.8  VectorParams1D=off
  Constant : Constant  Value=params.V
  Constant1 : Constant  Value=params.H
  Cw : Constant  Value=0.7  VectorParams1D=off
  Divide : Product  Inputs=*/
  Divide1 : Product  Inputs=*/
  Gain : Gain  Gain=1/100
  Gain1 : Gain  Gain=2*9.8100/4
  Minus : Sum  Inputs=-+
  Product : Product
  Product1 : Product
  Product2 : Product  Inputs=4
  Product3 : Product  Inputs=4
  Sqrt : Sqrt  SaturateOnIntegerOverflow=on
  Square : Math  Operator=square  SaturateOnIntegerOverflow=on
  Sum : Sum  Inputs=|++
  Sum1 : Sum  Inputs=|++
  c_i : Constant  Value=1.0032e+03  VectorParams1D=off
  R_a : Outport
  QV_i_e : Outport  Port=2
  wires:
  In Bus Element/1 -> Product2/3
  In Bus Element1/1 -> Gain/1
  wind_speed/1 -> Square/1
  Square/1 -> Product/1
  Cw/1 -> Product/2
  Product/1 -> Sum/2
  T_e/1 -> Minus/1, Divide/2
  <Tair>/1 -> Minus/2
  Minus/1 -> Product3/4, Abs/1
  Abs/1 -> Divide/1
  Constant1/1 -> Product1/2
  Divide/1 -> Product1/1
  Product1/1 -> Gain1/1
  Gain1/1 -> Sum/1
  Sum/1 -> Sqrt/1
  Sqrt/1 -> Product2/1
  Cd/1 -> Product2/2
  Product2/1 -> [Vdot]
  [Vdot] -> Divide1/1
  Constant/1 -> Divide1/2
  Divide1/1 -> R_a/1
  [Vdot] -> Product3/3
  rho_i/1 -> Product3/2
  c_i/1 -> Product3/1
  Product3/1 -> QV_i_e/1
  Gain/1 -> Sum1/1
  Sum1/1 -> Product2/4
  AR1/1 -> Sum1/2

== system HORTISIM/Climate/Models/Climate Model/Indoor Temperature Model/Heat Balance/nu compute ==
  In1 : Inport
  In2 : Inport  Port=2
  Constant : Constant
  Gain : Gain  Gain=1/100
  Product : Product
  Scope : Scope
  Sum : Sum  Inputs=|++
  Out1 : Outport
  wires:
  Gain/1 -> Product/2
  Product/1 -> Sum/1
  In2/1 -> Gain/1
  Constant/1 -> Sum/2
  In1/1 -> Product/1
  Sum/1 -> Out1/1, Scope/1

== system HORTISIM/Climate/Models/Climate Model/Indoor Temperature Model/Radiation Model/1-\alpha ==
  In1 : Inport
  Constant6 : Constant
  Minus : Sum  Inputs=+-
  Out1 : Outport
  wires:
  Minus/1 -> Out1/1
  In1/1 -> Minus/2
  Constant6/1 -> Minus/1

== system HORTISIM/Climate/Models/Climate Model/Indoor Temperature Model/Radiation Model/Subsystem ==
  A_f : Inport
  In2 : Inport  Port=2
  alpha_f : Inport  Port=3
  QS_i_tr : Inport  Port=4
  Divide : Product  Inputs=*/**
  Minus : Sum  Inputs=+-
  Out1 : Outport
  wires:
  QS_i_tr/1 -> Divide/4
  A_f/1 -> Divide/2, Minus/1
  Divide/1 -> Out1/1
  In2/1 -> Minus/2
  alpha_f/1 -> Divide/3
  Minus/1 -> Divide/1

== system HORTISIM/Climate/Models/Climate Model/Indoor Temperature Model/Radiation Model/tau_screen ==
  gamma : Inport
  screen : Inport  Port=2
  Constant3 : Constant
  Divide : Product  Inputs=**
  Gain : Gain  Gain=1/100
  Minus : Sum  Inputs=+-
  Out1 : Outport
  wires:
  gamma/1 -> Divide/1
  Divide/1 -> Gain/1
  Gain/1 -> Minus/2
  Minus/1 -> Out1/1
  screen/1 -> Divide/2
  Constant3/1 -> Minus/1

== system HORTISIM/Horticulture/Controls/Ferrtirrigation Controler/Irrigation Controler/If Action Subsystem/If Action Subsystem ==
  Action Port : ActionPort
  Constant : Constant  Value=0
  Out1 : Outport
  wires:
  Constant/1 -> Out1/1

== system HORTISIM/Horticulture/Controls/Ferrtirrigation Controler/Irrigation Controler/If Action Subsystem/If Action Subsystem1 ==
  Action Port : ActionPort
  Constant : Constant
  Out1 : Outport
  wires:
  Constant/1 -> Out1/1

== system HORTISIM/Horticulture/Models/Crop Grow/Crop Growth/Growth model/Growth Organs ==
  MC_photo : Inport
  MC_gro : Inport  Port=2
  MC_resp : Inport  Port=3
  MC_prune : Inport  Port=4
  harvest : Inport  Port=5
  Bus Creator : BusCreator  Inputs=4
  Bus Selector : BusSelector  OutputSignals=MC_buf_i,MC_fruit_i,MC_leaf_i,MC_stem_i
  Bus Selector1 : BusSelector  OutputSignals=MC_buf_fruit,MC_buf_leaf,MC_buf_stem
  Derivatives : MATLAB Function  TreatAsAtomicUnit=on
  dCdt : Outport
  wires:
  MC_prune/1 -> Derivatives/9(MC_leaf_prune)
  Derivatives/2(dC_fruit_dt) -> Bus Creator/2
  Derivatives/3(dC_leaf_dt) -> Bus Creator/3
  Derivatives/4(dC_stem_dt) -> Bus Creator/4
  Bus Creator/1 -> dCdt/1
  MC_resp/1 -> Bus Selector/1
  MC_gro/1 -> Bus Selector1/1
  MC_photo/1 -> Derivatives/1(MC_i_buf)
  Derivatives/1(dC_buff_dt) -> Bus Creator/1
  harvest/1 -> Derivatives/10(harvest)
  Bus Selector/1 -> [Buff_i]  "<MC_buf_i>"
  Bus Selector/4 -> [s_i]  "<MC_stem_i>"
  Bus Selector/2 -> [f_i]  "<MC_fruit_i>"
  Bus Selector/3 -> [l_i]  "<MC_leaf_i>"
  Bus Selector1/1 -> [Buff_f]  "<MC_buf_fruit>"
  Bus Selector1/2 -> [Buff_l]  "<MC_buf_leaf>"
  Bus Selector1/3 -> [Buff_s]  "<MC_buf_stem>"
  [s_i] -> Derivatives/8(MC_stem_i)
  [l_i] -> Derivatives/7(MC_leaf_i)
  [f_i] -> Derivatives/6(MC_fruit_i)
  [Buff_i] -> Derivatives/5(MC_buff_i)
  [Buff_s] -> Derivatives/4(MC_buf_stem)
  [Buff_l] -> Derivatives/3(MC_buf_leaf)
  [Buff_f] -> Derivatives/2(MC_buf_fruit)

== system HORTISIM/Horticulture/Models/Crop Grow/Crop Growth/Growth model/Nutrient Demand ==
  note: $kg\{Nutrients\}/(s\cdot m^2)$
  Crop : Inport
  Bus Selector : BusSelector  OutputSignals=Carbon.Cfruit,Carbon.Cleaf,Carbon.Cstem,Nutrients.Mass
  Gain : Gain  Gain=params.Chi_nutrients
  Gain1 : Gain  Gain=1e-3
  Minus : Sum  Inputs=+-
  Sum of Elements1 : Sum  Inputs=+++
  dNdt : Outport
  wires:
  Crop/1 -> Bus Selector/1
  Bus Selector/3 -> Sum of Elements1/3  "<Cstem>"
  Bus Selector/2 -> Sum of Elements1/2  "<Cleaf>"
  Bus Selector/1 -> Sum of Elements1/1  "<Cfruit>"
  Sum of Elements1/1 -> Gain/1
  Gain1/1 -> dNdt/1
  Bus Selector/4 -> Minus/2  "<Mass>"
  Gain/1 -> [chi_opt]
  [chi_opt] -> Minus/1
  Minus/1 -> Gain1/1

== system HORTISIM/Horticulture/Models/Crop Grow/Crop Growth/Growth model/Photosynthesis ==
  Crop : Inport
  " T_v" : Inport  Port=2
  "C_c " : Inport  Port=3
  rho_i : Inport  Port=4
  QS_v_VIS : Inport  Port=5
  Bus Selector1 : BusSelector  OutputSignals=Carbon.Cbuff,LAI,WaterPercent
  Constant : Constant  Value=0
  Constant1 : Constant  Value=params.A_v
  Constant2 : Constant  Value=params.C_buf_max
  Constant3 : Constant  Value=0.1
  Full Buffer Inibitor : $bdroot/Other  Functions/cumfun  SystemSampleTime=-1  VariantActivationTime=update diagram  Latency=0  AutoFrameSizeCalculation=off
  Gain : Gain  Gain=1/0.005
  Gain1 : Gain  Gain=4
  MATLAB Function : MATLAB Function  TreatAsAtomicUnit=on
  Max : MinMax  Function=max  Inputs=2
  Minus : Sum  Inputs=-+
  Minus1 : Sum  Inputs=+-
  Photosyntesis : MATLAB Function  TreatAsAtomicUnit=on
  Product : Product  Inputs=3
  Scope{,1..3} (4 alike) : Scope
  Scope4 : Scope  NumInputPorts=4
  cumfun : $bdroot/Other  Functions/cumfun  SystemSampleTime=-1  VariantActivationTime=update diagram  Latency=0  AutoFrameSizeCalculation=off
  MC_photo : Outport
  wires:
  Product/1 -> Scope2/1, MC_photo/1
  Photosyntesis/1(MC_i_buf) -> Product/3  "MC photo"
  Minus1/1 -> Gain1/1
  Constant3/1 -> Minus1/2
  [WP] -> Minus1/1
  Bus Selector1/3 -> [WP]  "<WaterPercent>"
  [CBuff] -> Minus/1  "Cbuff"
  Constant2/1 -> Minus/2
  Minus/1 -> Gain/1
  Gain/1 -> Full Buffer Inibitor/1
  Full Buffer Inibitor/1 -> Scope/1, Product/2  "H"
  Constant1/1 -> Photosyntesis/7(A_v)
  "C_c "/1 -> Photosyntesis/3(C_c)
  rho_i/1 -> Photosyntesis/4(rho_i)
  MATLAB Function/1(Gamma) -> Max/1
  Constant/1 -> Max/2
  Max/1 -> Scope3/1, Photosyntesis/6(Gamma)
  Crop/1 -> Bus Selector1/1
  " T_v"/1 -> MATLAB Function/1(T_v), Photosyntesis/5(T_v)
  QS_v_VIS/1 -> Scope1/1, Photosyntesis/1(QS_v_VIS)
  Bus Selector1/2 -> [LAI]  "<LAI>"
  [LAI] -> Photosyntesis/2(LAI)
  [LAI] -> MATLAB Function/2(LAI)
  Bus Selector1/1 -> [CBuff]  "<Cbuff>"
  Gain1/1 -> cumfun/1
  cumfun/1 -> Product/1
  Photosyntesis/2(PAR) -> Scope4/1
  Photosyntesis/3(P) -> Scope4/2
  Photosyntesis/4(Resp) -> Scope4/3
  Photosyntesis/5(C_stom) -> Scope4/4

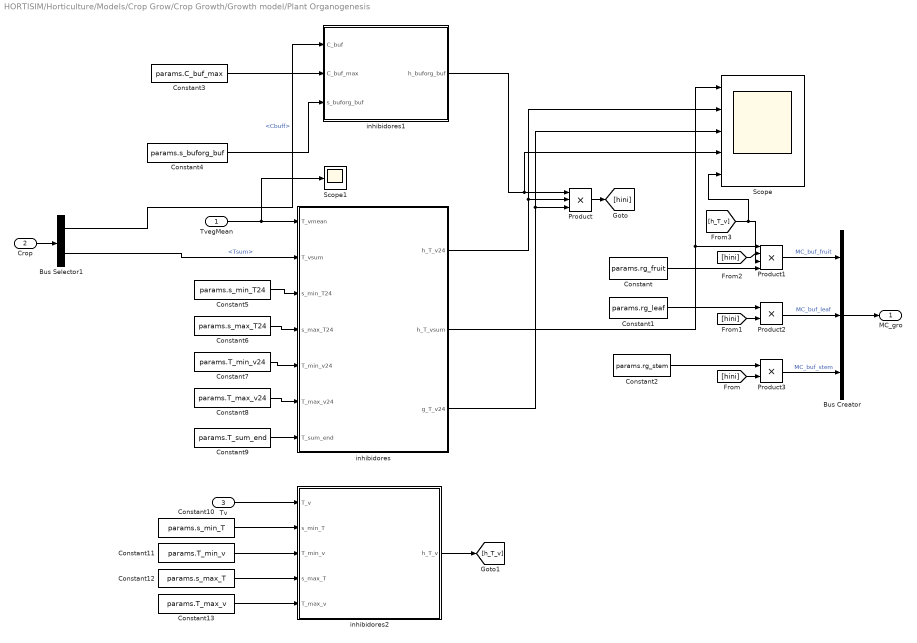
== system HORTISIM/Horticulture/Models/Crop Grow/Crop Growth/Growth model/Plant Organogenesis  ==
  TvegMean : Inport
  Crop : Inport  Port=2
  Tv : Inport  Port=3
  Bus Creator : BusCreator  Inputs=3
  Bus Selector1 : BusSelector  OutputSignals=Carbon.Cbuff,Tsum
  Constant : Constant  Value=params.rg_fruit
  Constant1 : Constant  Value=params.rg_leaf
  Constant10 : Constant  Value=params.s_min_T
  Constant11 : Constant  Value=params.T_min_v
  Constant12 : Constant  Value=params.s_max_T
  Constant13 : Constant  Value=params.T_max_v
  Constant2 : Constant  Value=params.rg_stem
  Constant3 : Constant  Value=params.C_buf_max
  Constant4 : Constant  Value=params.s_buforg_buf
  Constant5 : Constant  Value=params.s_min_T24
  Constant6 : Constant  Value=params.s_max_T24
  Constant7 : Constant  Value=params.T_min_v24
  Constant8 : Constant  Value=params.T_max_v24
  Constant9 : Constant  Value=params.T_sum_end
  Product : Product  Inputs=3
  Product1 : Product  Inputs=4
  Product2 : Product
  Product3 : Product
  Scope : Scope  NumInputPorts=5
  Scope1 : Scope
  inhibidores : MATLAB Function  TreatAsAtomicUnit=on
  inhibidores1 : MATLAB Function  TreatAsAtomicUnit=on
  inhibidores2 : MATLAB Function  TreatAsAtomicUnit=on
  MC_gro : Outport
  wires:
  [hini] -> Product1/2
  [hini] -> Product2/2
  [hini] -> Product3/2
  Product/1 -> [hini]
  Constant2/1 -> Product3/1
  Constant1/1 -> Product2/1
  inhibidores/2(h_T_vsum) -> Scope/1, Product1/1
  Constant/1 -> Product1/4
  inhibidores1/1(h_buforg_buf) -> Scope/4, Product/1
  Constant9/1 -> inhibidores/7(T_sum_end)
  Constant8/1 -> inhibidores/6(T_max_v24)
  Constant7/1 -> inhibidores/5(T_min_v24)
  Constant6/1 -> inhibidores/4(s_max_T24)
  Constant5/1 -> inhibidores/3(s_min_T24)
  Constant3/1 -> inhibidores1/2(C_buf_max)
  Crop/1 -> Bus Selector1/1
  Bus Creator/1 -> MC_gro/1
  inhibidores/1(h_T_v24) -> Scope/2, Product/2
  inhibidores/3(g_T_v24) -> Scope/3, Product/3
  Product1/1 -> Bus Creator/1  "MC_buf_fruit"
  Product2/1 -> Bus Creator/2  "MC_buf_leaf"
  Product3/1 -> Bus Creator/3  "MC_buf_stem"
  Bus Selector1/2 -> inhibidores/2(T_vsum)  "<Tsum>"
  TvegMean/1 -> Scope1/1, inhibidores/1(T_vmean)
  Bus Selector1/1 -> inhibidores1/1(C_buf)  "<Cbuff>"
  Constant4/1 -> inhibidores1/3(s_buforg_buf)
  Tv/1 -> inhibidores2/1(T_v)
  Constant10/1 -> inhibidores2/2(s_min_T)
  Constant11/1 -> inhibidores2/3(T_min_v)
  Constant12/1 -> inhibidores2/4(s_max_T)
  Constant13/1 -> inhibidores2/5(T_max_v)
  inhibidores2/1(h_T_v) -> [h_T_v]
  [h_T_v] -> Scope/5, Product1/3

== system HORTISIM/Horticulture/Models/Crop Grow/Crop Growth/Growth model/Relative Growth ==
  Crop : Inport
  MC_leaf_prune : Inport  Port=2
  dCdt : Inport  Port=3
  harvest : Inport  Port=4
  Bus Selector : BusSelector  OutputSignals=Carbon.Cbuff,Carbon.Cfruit,Carbon.Cleaf,Relative.Rfruit,Relative.Rleaf,Relative.Rstem
  Bus Selector1 : BusSelector  OutputSignals=dC_fruit_dt,dC_fruit_dt,dC_fruit_dt
  Relative Growth : MATLAB Function  TreatAsAtomicUnit=on
  Vector Concatenate : Concatenate  NumInputs=3
  dRdt : Outport
  wires:
  Relative Growth/2(dR_leaf_dt) -> Vector Concatenate/2
  Relative Growth/3(dR_stem_dt) -> Vector Concatenate/3
  Relative Growth/1(dR_fruit_dt) -> Vector Concatenate/1
  MC_leaf_prune/1 -> Relative Growth/10(MC_leaf_prune)
  Vector Concatenate/1 -> dRdt/1
  Crop/1 -> Bus Selector/1
  dCdt/1 -> Bus Selector1/1
  Bus Selector1/2 -> Relative Growth/2(dC_leaf_dt)  "<dC_fruit_dt>"
  Bus Selector1/1 -> Relative Growth/1(dC_fruit_dt)  "<dC_fruit_dt>"
  Bus Selector1/3 -> Relative Growth/3(dC_stem_dt)  "<dC_fruit_dt>"
  Bus Selector/6 -> Relative Growth/9(R_stem)  "<Rstem>"
  Bus Selector/5 -> Relative Growth/8(R_leaf)  "<Rleaf>"
  Bus Selector/4 -> Relative Growth/7(R_fruit)  "<Rfruit>"
  Bus Selector/3 -> Relative Growth/6(C_stem)  "<Cleaf>"
  Bus Selector/2 -> Relative Growth/5(C_leaf)  "<Cfruit>"
  Bus Selector/1 -> Relative Growth/4(C_fruit)  "<Cbuff>"
  harvest/1 -> Relative Growth/11(harvest)
